simulink model "LabFabSim2022a__2_9_2023_AllAttacks_"  (R2022a)
settings: Solver=VariableStepAuto  StartTime=0.0  StopTime=5500000  RelTol=1e-3  EnableMultiTasking=on
model workspace (MAT data in the model file):
  JsonData : timetable (value not decoded)
  M : Simulink.Parameter (value not decoded)
  ROS_trigger = 0
  SL_ROS_VariableLengthArrays_MaxSizes : object (value not decoded)
undefined symbols (not defined in the file): DOS, DOSinitGen, DTP, DTPGen, DTPInitGen, EmptyLocFound, InitCobot, InitCobotReturn, InitializeSLD, InitLEGO, InitVGRproc2, m, MC, MCGen, MCInitGen, MO, MOGen, MOInitGen, n, NetScan, NetScanInitGen, Spying, SpyingInitGen, WS, WSGen, WSInitGen
libraries: sldelib x6
(part 4 of 4)

== system LabFabSim2022a__2_9_2023_AllAttacks_/Spying/Spying ==
  Spying : TriggerPort  TriggerType=function-call  IsSimulinkFunction=on  FunctionName=Spying  VariantControl=(inherit)
  Message Send : Send  OutputPortMessageModes=m
  u : ArgIn  DisableCoverage=on  ArgumentName=u
  Out1 : Outport
  wires:
  u/1 -> Message Send/1
  Message Send/1 -> Out1/1

== system LabFabSim2022a__2_9_2023_AllAttacks_/Spying/Subsystem1 ==
  Constant : Constant
  Out1 : Outport
  wires:
  Constant/1 -> Out1/1

== system LabFabSim2022a__2_9_2023_AllAttacks_/VGR Moves to HBW (MO)/Simulink Function ==
  BinSupplied : TriggerPort  TriggerType=function-call  IsSimulinkFunction=on  FunctionName=BinSupplied  VariantControl=(inherit)
  Constant : Constant
  Message Send : Send  OutputPortMessageModes=m
  Out1 : Outport
  wires:
  Constant/1 -> Message Send/1
  Message Send/1 -> Out1/1

== system LabFabSim2022a__2_9_2023_AllAttacks_/VGR Moves to HBW (MO)/Simulink Function2 ==
  MO_Router : TriggerPort  TriggerType=function-call  IsSimulinkFunction=on  FunctionName=MO_Router  VariantControl=(inherit)
  Constant : Constant  Value=2
  Constant1 : Constant
  Switch : Switch  Threshold=2  ZeroCross=off  SaturateOnIntegerOverflow=off  InputSameDT=off
  u : ArgIn  DisableCoverage=on  ArgumentName=u
  Out1 : Outport
  wires:
  u/1 -> Switch/2
  Switch/1 -> Out1/1
  Constant1/1 -> Switch/1
  Constant/1 -> Switch/3

== system LabFabSim2022a__2_9_2023_AllAttacks_/VGR_Proc1 (WS & MC)/Simulink Function ==
  MPS_Initialize() : TriggerPort  TriggerType=function-call  IsSimulinkFunction=on  FunctionName=MPS_Initialize  VariantControl=(inherit)
  Constant : Constant
  Message Send : Send  OutputPortMessageModes=m
  Out1 : Outport
  wires:
  Constant/1 -> Message Send/1
  Message Send/1 -> Out1/1

== system LabFabSim2022a__2_9_2023_AllAttacks_/VGR_Proc1 (WS & MC)/Simulink Function1 ==
  MC_Router : TriggerPort  TriggerType=function-call  IsSimulinkFunction=on  FunctionName=MC_Router  VariantControl=(inherit)
  Constant : Constant  Value=2
  Constant1 : Constant
  Switch : Switch  Threshold=2  ZeroCross=off  SaturateOnIntegerOverflow=off  InputSameDT=off
  u : ArgIn  DisableCoverage=on  ArgumentName=u
  Out1 : Outport
  wires:
  u/1 -> Switch/2
  Switch/1 -> Out1/1
  Constant1/1 -> Switch/1
  Constant/1 -> Switch/3

== system LabFabSim2022a__2_9_2023_AllAttacks_/VGR_Proc1 (WS & MC)/Simulink Function2 ==
  WS_Router : TriggerPort  TriggerType=function-call  IsSimulinkFunction=on  FunctionName=WS_Router  VariantControl=(inherit)
  Constant : Constant  Value=2
  Constant1 : Constant
  Switch : Switch  Threshold=2  ZeroCross=off  SaturateOnIntegerOverflow=off  InputSameDT=off
  u : ArgIn  DisableCoverage=on  ArgumentName=u
  Out1 : Outport
  wires:
  u/1 -> Switch/2
  Switch/1 -> Out1/1
  Constant1/1 -> Switch/1
  Constant/1 -> Switch/3

== system LabFabSim2022a__2_9_2023_AllAttacks_/VGR_Proc2 (Spying)/Simulink Function ==
  InitCobot() : TriggerPort  TriggerType=function-call  IsSimulinkFunction=on  FunctionName=InitCobot  VariantControl=(inherit)
  Constant : Constant
  Message Send : Send  OutputPortMessageModes=m
  Out1 : Outport
  wires:
  Constant/1 -> Message Send/1
  Message Send/1 -> Out1/1

== system LabFabSim2022a__2_9_2023_AllAttacks_/VGR_Proc2 (Spying)/Simulink Function2 ==
  Spying_Router : TriggerPort  TriggerType=function-call  IsSimulinkFunction=on  FunctionName=Spying_Router  VariantControl=(inherit)
  Constant : Constant  Value=2
  Constant1 : Constant
  Switch : Switch  Threshold=2  ZeroCross=off  SaturateOnIntegerOverflow=off  InputSameDT=off
  u : ArgIn  DisableCoverage=on  ArgumentName=u
  Out1 : Outport
  wires:
  u/1 -> Switch/2
  Switch/1 -> Out1/1
  Constant1/1 -> Switch/1
  Constant/1 -> Switch/3

== system LabFabSim2022a__2_9_2023_AllAttacks_/VGR_Proc3 (Ramp)/Simulink Function ==
  EmptyLocFound() : TriggerPort  TriggerType=function-call  IsSimulinkFunction=on  FunctionName=EmptyLocFound  VariantControl=(inherit)
  Constant : Constant
  Message Send : Send  OutputPortMessageModes=m
  Out1 : Outport
  wires:
  Constant/1 -> Message Send/1
  Message Send/1 -> Out1/1

== system LabFabSim2022a__2_9_2023_AllAttacks_/WrongSetup (WS)/InitWrongSetup ==
  note: On Entry: Generate 1 Wrong Setup attack entities
  Entity Generator1 : EntityGenerator  InputPortMessageModes=m  OutputPortMessageModes=m  GenerationMethod=Event-based  Period=inf  AttributeName=data  EntityType=Structured  EntityTypeName=InitWS
      settings: InputPortMap=u0
  Entity Terminator2 : EntityTerminator  InputPortMessageModes=m  EntryAction=WSGen();  NumberEntitiesArrived=on
      settings: OutputPortMap=o0
  Simulink Function2 : Subsystem  TreatAsAtomicUnit=on
  Subsystem2 : Subsystem
  Out1 : Outport
  wires:
  Subsystem2/1(Out1) -> Simulink Function2/1(In1)
  Simulink Function2/1(Out1) -> Entity Generator1/1
  Entity Terminator2/1 -> Out1/1
  Entity Generator1/1 -> Entity Terminator2/1

== system LabFabSim2022a__2_9_2023_AllAttacks_/WrongSetup (WS)/Simulink Function1 ==
  In1 : Inport
  WSGen : TriggerPort  TriggerType=function-call  IsSimulinkFunction=on  FunctionName=WSGen  VariantControl=(inherit)
  Message Send : Send  OutputPortMessageModes=m
  Out1 : Outport
  wires:
  Message Send/1 -> Out1/1
  In1/1 -> Message Send/1

== system LabFabSim2022a__2_9_2023_AllAttacks_/WrongSetup (WS)/Subsystem1 ==
  Constant : Constant
  Out1 : Outport
  wires:
  Constant/1 -> Out1/1

== system LabFabSim2022a__2_9_2023_AllAttacks_/WrongSetup (WS)/Wrong Setup ==
  WS : TriggerPort  TriggerType=function-call  IsSimulinkFunction=on  FunctionName=WS  VariantControl=(inherit)
  Message Send : Send  OutputPortMessageModes=m
  u : ArgIn  DisableCoverage=on  ArgumentName=u
  Out1 : Outport
  wires:
  u/1 -> Message Send/1
  Message Send/1 -> Out1/1

== system LabFabSim2022a__2_9_2023_AllAttacks_/DOS/InitDOS/Simulink Function2 ==
  In1 : Inport
  DOSinitGen : TriggerPort  TriggerType=function-call  IsSimulinkFunction=on  FunctionName=DOSinitGen  VariantControl=(inherit)
  Message Send : Send  OutputPortMessageModes=m
  Out1 : Outport
  wires:
  Message Send/1 -> Out1/1
  In1/1 -> Message Send/1

== system LabFabSim2022a__2_9_2023_AllAttacks_/DOS/InitDOS/Subsystem2 ==
  Constant : Constant
  Out1 : Outport
  wires:
  Constant/1 -> Out1/1

== system LabFabSim2022a__2_9_2023_AllAttacks_/DataTypesProbing (DTP)/InitDataTypesProbing/Simulink Function2 ==
  In1 : Inport
  DTPInitGen : TriggerPort  TriggerType=function-call  IsSimulinkFunction=on  FunctionName=DTPInitGen  VariantControl=(inherit)
  Message Send : Send  OutputPortMessageModes=m
  Out1 : Outport
  wires:
  Message Send/1 -> Out1/1
  In1/1 -> Message Send/1

== system LabFabSim2022a__2_9_2023_AllAttacks_/DataTypesProbing (DTP)/InitDataTypesProbing/Subsystem2 ==
  Constant : Constant
  Out1 : Outport
  wires:
  Constant/1 -> Out1/1

== system LabFabSim2022a__2_9_2023_AllAttacks_/MaliciousControl (MC)/InitMaliciousControl/Simulink Function2 ==
  In1 : Inport
  MCInitGen : TriggerPort  TriggerType=function-call  IsSimulinkFunction=on  FunctionName=MCInitGen  VariantControl=(inherit)
  Message Send : Send  OutputPortMessageModes=m
  Out1 : Outport
  wires:
  Message Send/1 -> Out1/1
  In1/1 -> Message Send/1

== system LabFabSim2022a__2_9_2023_AllAttacks_/MaliciousControl (MC)/InitMaliciousControl/Subsystem2 ==
  Constant : Constant
  Out1 : Outport
  wires:
  Constant/1 -> Out1/1

== system LabFabSim2022a__2_9_2023_AllAttacks_/MaliciousOperation (MO)/InitMaliciousOperation/Simulink Function2 ==
  In1 : Inport
  MOInitGen : TriggerPort  TriggerType=function-call  IsSimulinkFunction=on  FunctionName=MOInitGen  VariantControl=(inherit)
  Message Send : Send  OutputPortMessageModes=m
  Out1 : Outport
  wires:
  Message Send/1 -> Out1/1
  In1/1 -> Message Send/1

== system LabFabSim2022a__2_9_2023_AllAttacks_/MaliciousOperation (MO)/InitMaliciousOperation/Subsystem2 ==
  Constant : Constant
  Out1 : Outport
  wires:
  Constant/1 -> Out1/1

== system LabFabSim2022a__2_9_2023_AllAttacks_/NetworkScan/InitNetScan/Simulink Function2 ==
  In1 : Inport
  NetScanInitGen : TriggerPort  TriggerType=function-call  IsSimulinkFunction=on  FunctionName=NetScanInitGen  VariantControl=(inherit)
  Message Send : Send  OutputPortMessageModes=m
  Out1 : Outport
  wires:
  Message Send/1 -> Out1/1
  In1/1 -> Message Send/1

== system LabFabSim2022a__2_9_2023_AllAttacks_/NetworkScan/InitNetScan/Subsystem2 ==
  Constant : Constant
  Out1 : Outport
  wires:
  Constant/1 -> Out1/1

== system LabFabSim2022a__2_9_2023_AllAttacks_/Spying/InitSpying/Simulink Function2 ==
  In1 : Inport
  SpyingInitGen : TriggerPort  TriggerType=function-call  IsSimulinkFunction=on  FunctionName=SpyingInitGen  VariantControl=(inherit)
  Message Send : Send  OutputPortMessageModes=m
  Out1 : Outport
  wires:
  Message Send/1 -> Out1/1
  In1/1 -> Message Send/1

== system LabFabSim2022a__2_9_2023_AllAttacks_/Spying/InitSpying/Subsystem2 ==
  Constant : Constant
  Out1 : Outport
  wires:
  Constant/1 -> Out1/1

== system LabFabSim2022a__2_9_2023_AllAttacks_/WrongSetup (WS)/InitWrongSetup/Simulink Function2 ==
  In1 : Inport
  WSInitGen : TriggerPort  TriggerType=function-call  IsSimulinkFunction=on  FunctionName=WSInitGen  VariantControl=(inherit)
  Message Send : Send  OutputPortMessageModes=m
  Out1 : Outport
  wires:
  Message Send/1 -> Out1/1
  In1/1 -> Message Send/1

== system LabFabSim2022a__2_9_2023_AllAttacks_/WrongSetup (WS)/InitWrongSetup/Subsystem2 ==
  Constant : Constant
  Out1 : Outport
  wires:
  Constant/1 -> Out1/1
